simulink model "trajectory_with_control"  (R2017a)
settings: Solver=ode4  StartTime=0.0  StopTime=250  FixedStep=0.01  RelTol=1e-3
libraries: simulink x1
settings Model: Creator=Alex  LastModifiedBy=Alex

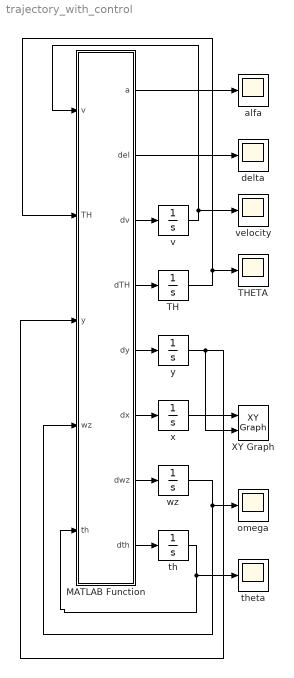
== system trajectory_with_control ==
  MATLAB Function : MATLAB Function  TreatAsAtomicUnit=on
  TH : Integrator
  THETA : Scope
  XY Graph : simulink/Sinks/XY Graph  xmin=0  xmax=25000  ymin=0  ymax=8000  st=-1
  alfa : Scope
  delta : Scope
  omega : Scope
  th : Integrator
  theta : Scope
  v : Integrator  InitialCondition=159.44
  velocity : Scope
  wz : Integrator
  x : Integrator
  y : Integrator  InitialCondition=3800
  wires:
  v/1 -> velocity/1, MATLAB Function/1(v)
  MATLAB Function/4(dTH) -> TH/1
  y/1 -> XY Graph/2, MATLAB Function/3(y)
  MATLAB Function/6(dx) -> x/1
  MATLAB Function/3(dv) -> v/1
  MATLAB Function/5(dy) -> y/1
  x/1 -> XY Graph/1
  MATLAB Function/7(dwz) -> wz/1
  MATLAB Function/8(dth) -> th/1
  wz/1 -> omega/1, MATLAB Function/4(wz)
  th/1 -> theta/1, MATLAB Function/5(th)
  TH/1 -> MATLAB Function/2(TH), THETA/1
  MATLAB Function/2(del) -> delta/1
  MATLAB Function/1(a) -> alfa/1

== matlab function trajectory_with_control/MATLAB Function ==
  data: a output; del output; dv output; dTH output; dy output; dx output; v input; TH input; y input; wz input; th input; dwz output; dth output
function [a, del, dv, dTH, dy, dx,    dwz, dth] = fcn(v, TH, y,    wz, th)

m = 4000;
R = 9000;

v_i = [111.11 159.44 205.56];
Cx_i = [0.090 0.092 0.096];
Cy_i = [0.147 0.149 0.151];

if v < v_i(1) || v > v_i(end)
    
    Cx = interp1(v_i, Cx_i, v, 'linear', 'extrap');
    Cy = interp1(v_i, Cy_i, v, 'linear', 'extrap');
   
else
    Cx = interp1(v_i, Cx_i, v, 'linear');
    Cy = interp1(v_i, Cy_i, v, 'linear');
    
end

% Cx = 0.1;
% Cy = 0.3;
S = 16.1;
ro = 1.22*exp(-y/10000);
q = (ro * v^2) / 2;

X = Cx * q * S;
Y = Cy * q * S;

g = 9.81;
G = m*g;

%a = 3;


%задающий тангаж:
%u = 3;
u = 3 * pi/180;

%коэффициенты:
I1 = -10000; I2 = -1500;

a11 = 0.032; a12 = 0.04; a13 = 0.021; a42 = 0.033;
%a11 = 0.031640078559898 * 180/pi; a12 = 0.040077432842537 * 180/pi; a13 = 0.021515253420731 * 180/pi;

%в радианах:
a = th - TH;
dv = (R - X - G*sin(TH)) / m;
%dTH = (R*a - G*cos(TH) + Y) / m / v;
dTH = a42*a;
dx = v*cos(TH);
dy = v*sin(TH);

del = I1*(u - th) - I2*wz;
dwz = -a12*a - a11*wz - a13*del;
dth = wz;

%в градусах:
% a = th - TH;
% dv = (R - X - G*sind(TH)) / m;
% dTH = (R*a - G*cosd(TH) + Y) / m / v;
% dx = v*cosd(TH);
% dy = v*sind(TH);
% 
% del = I1*(u - th) - I2*wz;
% dwz = -a12*a - a11*wz - a13*del;
% dth = wz;
